simulink model "score"  (R2021a)
settings: Solver=VariableStepAuto  StartTime=0.0  StopTime=1000  RelTol=1e-6
model workspace (MAT data in the model file):
  Ts = 10
  amp = 1.1
  capacity = 100
  initial_available = 43
  limit = 0.052
  lowSpaceRatio = 0.8
  nums1 = [0.333333333333 0.266666666667 0.2 0.133333333333 0.0666666666667]
  tolerate = 1752510
undefined symbols (not defined in the file or in its folder): DiscIntNeverNeededParam, hma_dens, hma_nums
libraries: pingcap x4
settings Model: Creator=tongjian  LastModifiedBy=tongjian

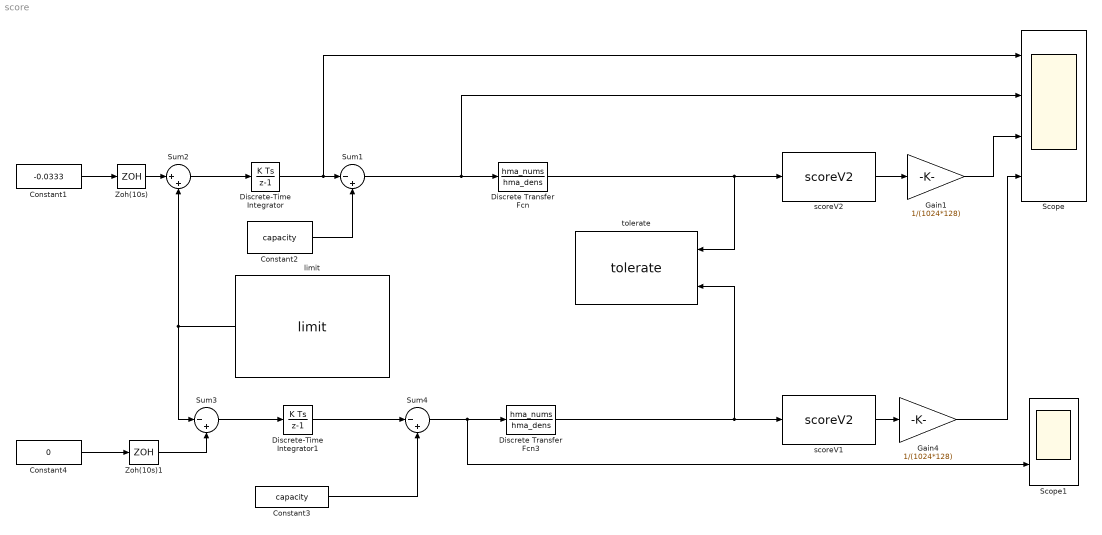
== system score ==
  Constant1 : Constant  Value=-0.0333
  Constant2 : Constant  Value=capacity
  Constant3 : Constant  Value=capacity
  Constant4 : Constant  Value=0
  Discrete Transfer Fcn : DiscreteTransferFcn  Numerator=hma_nums  Denominator=hma_dens  InitialStates=initial_available  SampleTime=Ts
  Discrete Transfer Fcn3 : DiscreteTransferFcn  Numerator=hma_nums  Denominator=hma_dens  InitialStates=initial_available  SampleTime=Ts
  Discrete-Time Integrator : DiscreteIntegrator  gainval=Ts  InitialCondition=initial_available  SampleTime=10  ICPrevOutput=DiscIntNeverNeededParam  ICPrevScaledInput=DiscIntNeverNeededParam
  Discrete-Time Integrator1 : DiscreteIntegrator  gainval=Ts  InitialCondition=initial_available  SampleTime=10  ICPrevOutput=DiscIntNeverNeededParam  ICPrevScaledInput=DiscIntNeverNeededParam
  Gain1 : Gain  Gain=1/(1024*128)
  Gain4 : Gain  Gain=1/(1024*128)
  Scope : Scope  NumInputPorts=4
  Scope1 : Scope  NumInputPorts=2
  Sum1 : Sum  Inputs=|-+
  Sum2 : Sum  Inputs=|++
  Sum3 : Sum  Inputs=|-+
  Sum4 : Sum  Inputs=|-+
  Zoh(10s) : ZeroOrderHold  Description=Zoh(10s)  SampleTime=10
  Zoh(10s)1 : ZeroOrderHold  Description=Zoh(10s)  SampleTime=10
  limit : pingcap/limit  g_limit=tolerate  g_value=limit
  scoreV1 : pingcap/scoreV2  g_lowSpaceRatio=lowSpaceRatio  g_amp=amp  g_capacity=capacity
  scoreV2 : pingcap/scoreV2  g_lowSpaceRatio=lowSpaceRatio  g_amp=amp  g_capacity=capacity
  tolerate : pingcap/tolerate  g_tolerateSize=0
  wires:
  Zoh(10s)/1 -> Sum2/1
  Discrete-Time Integrator/1 -> Scope/1, Sum1/1
  Sum2/1 -> Discrete-Time Integrator/1
  Constant2/1 -> Sum1/2
  Sum1/1 -> Scope/2, Discrete Transfer Fcn/1
  Discrete Transfer Fcn/1 -> tolerate/1, scoreV2/1
  scoreV2/1 -> Gain1/1
  Discrete Transfer Fcn3/1 -> tolerate/2, scoreV1/1
  scoreV1/1 -> Gain4/1
  Constant3/1 -> Sum4/2
  Constant4/1 -> Zoh(10s)1/1
  Zoh(10s)1/1 -> Sum3/2
  Sum3/1 -> Discrete-Time Integrator1/1
  Sum4/1 -> Scope1/2, Discrete Transfer Fcn3/1
  limit/1 -> Sum2/2, Sum3/1
  Constant1/1 -> Zoh(10s)/1
  Gain1/1 -> Scope/3
  Gain4/1 -> Scope/4
  Discrete-Time Integrator1/1 -> Sum4/1
